simulink model "Exp01_06_Single_Phase_Transformer"  (R2023a)
settings: Solver=VariableStepAuto  StartTime=0.0  StopTime=.02  RelTol=1e-3
libraries: nesl_utility x13, fl_lib x8, ee_lib x8, spsPowerLib x2, spsRMSLib x2, spspowerguiLib x1
settings Model: Creator=dougs  LastModifiedBy=rafin
settings SolverCC: AlgebraicLoopSolver=TrustRegion
settings DebuggingCC: UnconnectedInputMsg=warning  UnconnectedOutputMsg=warning  UnconnectedLineMsg=warning
settings ModelReferenceCC: EnableRefExpFcnMdlSchedulingChecks=on
settings RTWCC: DLArmComputeVersion=19.05

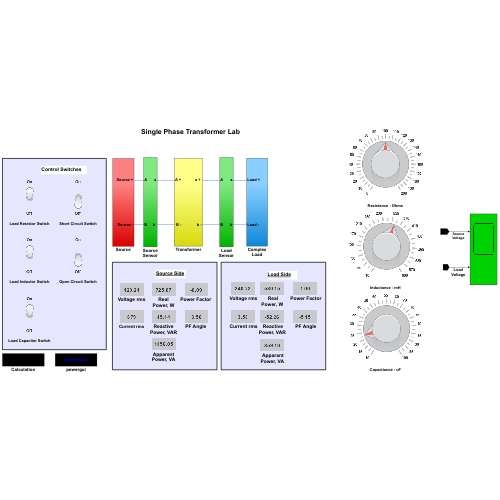
[thumbnail: Simulink's stored preview of the top-level diagram]
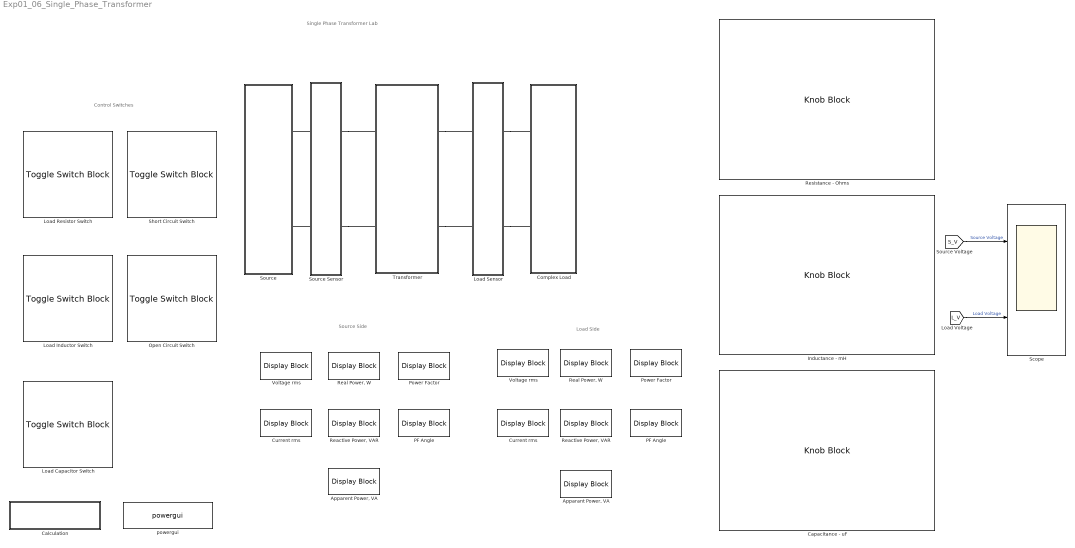
== system Exp01_06_Single_Phase_Transformer ==
  note: Control Switches
  note: Source Side
  note: Single Phase Transformer Lab
  note: Load Side
  " Apparant Power, VA" : DisplayBlock  LabelPosition=Hide  Format=bank  Transparency=1
  " Current rms" : DisplayBlock  LabelPosition=Hide  Format=bank  Transparency=1
  " PF Angle" : DisplayBlock  LabelPosition=Hide  Format=bank  Transparency=1
  " Power Factor" : DisplayBlock  LabelPosition=Hide  Format=bank  Transparency=1
  " Reactive Power, VAR" : DisplayBlock  LabelPosition=Hide  Format=bank  Transparency=1
  " Real Power, W" : DisplayBlock  LabelPosition=Hide  Format=bank  Transparency=1
  " Voltage rms" : DisplayBlock  LabelPosition=Hide  Format=bank  Transparency=1
  "Apparent Power, VA" : DisplayBlock  LabelPosition=Hide  Format=bank  Transparency=1
  Calculation : Subsystem
  Capacitance - uF : KnobBlock  LabelPosition=Hide  ScaleMin=10
  Complex Load : Subsystem
  Current rms : DisplayBlock  LabelPosition=Hide  Format=bank  Transparency=1
  Inductance - mH : KnobBlock  LabelPosition=Hide  ScaleMin=10  ScaleMax=600
  Load Sensor : Subsystem
  Load Capacitor Switch : ToggleSwitchBlock  LabelPosition=Hide
      settings: Values={{'Off', 'On'}, [0 2]}
  Load Inductor Switch : ToggleSwitchBlock  LabelPosition=Hide
      settings: Values={{'Off', 'On'}, [0 2]}
  Load Resistor Switch : ToggleSwitchBlock  LabelPosition=Hide
      settings: Values={{'Off', 'On'}, [0 2]}
  Open Circuit Switch : ToggleSwitchBlock  LabelPosition=Hide
      settings: Values={{'Off', 'On'}, [2 -2]}
  "PF Angle " : DisplayBlock  LabelPosition=Hide  Format=bank  Transparency=1
  "Power Factor " : DisplayBlock  LabelPosition=Hide  Format=bank  Transparency=1
  "Reactive Power, VAR" : DisplayBlock  LabelPosition=Hide  Format=bank  Transparency=1
  "Real Power, W" : DisplayBlock  LabelPosition=Hide  Format=bank  Transparency=1
  Resistance - Ohms : KnobBlock  LabelPosition=Hide  ScaleMax=200  TickInterval=10
  Scope : Scope  NumInputPorts=2
  Short Circuit Switch : ToggleSwitchBlock  LabelPosition=Hide
      settings: Values={{'Off', 'On'}, [0 2]}
  Source : Subsystem
      settings: PortSchema="{\"entries\":[{\"content\":{\"sides\":[{\"content\":{\"connectorIds\":[]},\"type\":\"ConnectorPlacement.EquallySpacedRectSide\",\"uuid\":\"e57deccf-7da9-425e-89f3-6f5e29807383\"},{\"content\":{\"connectorIds\":[],\"side\":\"RIGHT\"},\"type\":\"ConnectorPlacement.EquallySpacedRectSide\",\"uuid\":\"3e2a9798-8009-4f77-a4c3-5ae74279a04d\"},{\"content\":{\"connectorIds\":[],\"side\":\"TOP\"},\"type\":\"ConnectorPlacement.EquallySpacedRectSide\",\"uuid\":\"7dc73e5d-785d-4517-961f-ba0b2f479572\"},{\"content\":{\"connectorIds\":[\"RConn1\",\"RConn2\"],\"side\":\"BOTTOM\"},\"type\":\"ConnectorPlacement.EquallySpacedRectSide\",\"uuid\":\"c1959ef5-3070-4240-ae81-20c207906e41\"}]},\"type\":\"ConnectorPlacement.EquallySpacedConnector\",\"uuid\":\"719f97bd-ed7f-4cfa-8d10-4518bed19cde\"}],\"packageUris\":[\"http://schema.mathworks.com/mf0/Connector/R2020b\"],\"version\":\"1.0\"}"
  Source Sensor : Subsystem
  Transformer : Subsystem
  Voltage rms : DisplayBlock  LabelPosition=Hide  Format=bank  Transparency=1
  powergui : spspowerguiLib/powergui  Priority=1  SimulationMode=Continuous  SampleTime=50e-6  frequency=60  Iterations=50  frequencyindice=60  Pbase=100e6  ErrMax=1e-4  UnitsV=kV  UnitsW=MW  buscounter=0  FunctionMessages=off  echomessages=off  EnableUseOfTLC=off  CurrentSourceSwitches=off  DisableSnubberDevices=off  DisableRonSwitches=off  DisableVfSwitches=off  DisplayEquations=off  AutomaticDiscreteSolvers=off  SolverType=Tustin/Backward Euler (TBE)  Interpol=off  ExternalGateDelay=off  methode=off  Ts=100  x0status=blocks  SPID=on  SwTol=0  HookPort=off  NonlinearTolerance=1e-4  nMaxIteration=100  ContinueOnMaxIteration=off  RestoreLinks=warning  ResistiveCurrentMeasurement=off  Frange=[0:2:500]  Ylog=off  Xlog=on  ShowGrid=off  save=off  variable=ZData  structure=0  ZoomFFT=off  StartTime=0.0  cycles=1  DisplayStyle=1  fundamental=60  FreqAxis=off  MaxFrequency=1000  frequencyindicesteady=1  RmsSteady=1  display=off
  wires:
  [S_V] -> Scope/1  "Source Voltage"
  [L_V] -> Scope/2  "Load Voltage"
  connections:
  Load Sensor/RConn2 -- Complex Load/LConn2
  Load Sensor/RConn1 -- Complex Load/LConn1
  Transformer/RConn2 -- Load Sensor/LConn2
  Transformer/RConn1 -- Load Sensor/LConn1
  Source Sensor/RConn1 -- Transformer/LConn1
  Source Sensor/RConn2 -- Transformer/LConn2
  Source Sensor/LConn1 -- Source/RConn1
  Source Sensor/LConn2 -- Source/RConn2

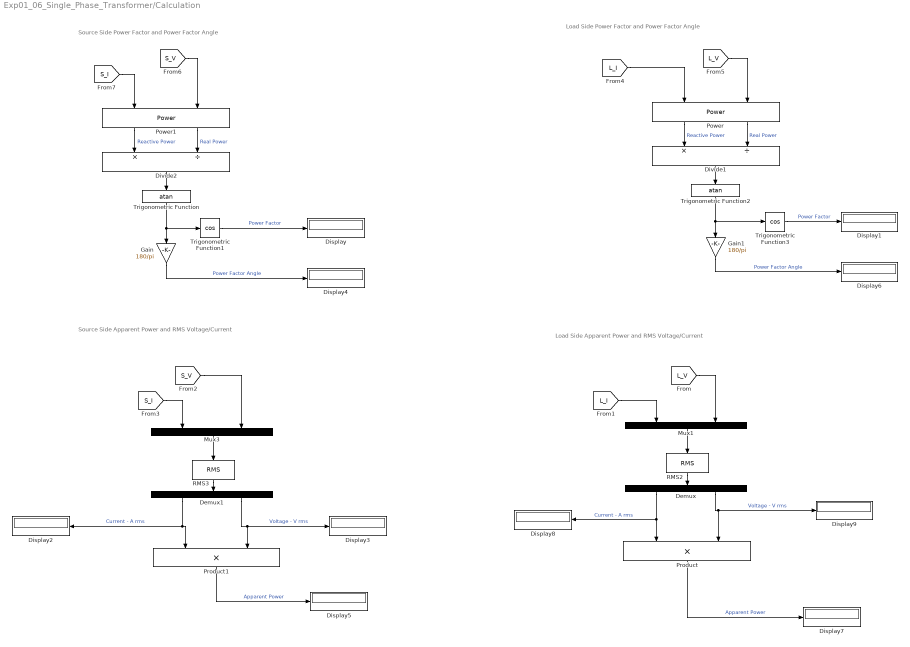
== system Exp01_06_Single_Phase_Transformer/Calculation ==
  note: Source Side Power Factor and Power Factor Angle
  note: Source Side Apparent Power and RMS Voltage/Current
  note: Load Side Power Factor and Power Factor Angle
  note: Load Side Apparent Power and RMS Voltage/Current
  Demux : Demux  Outputs=2
  Demux1 : Demux  Outputs=2
  Display{,1..9} (10 alike) : Display
  Divide1 : Product  Inputs=*/
  Divide2 : Product  Inputs=*/
  Gain : Gain  Gain=180/pi
  Gain1 : Gain  Gain=180/pi
  Mux1 : Mux  Inputs=2
  Mux3 : Mux  Inputs=2
  Power : spsPowerLib/Power  Freq=60  Vinit=[1, 0]  Iinit=[1, 0]  Ts=0
  Power1 : spsPowerLib/Power  Freq=60  Vinit=[1, 0]  Iinit=[1, 0]  Ts=0
  Product : Product
  Product1 : Product
  RMS2 : spsRMSLib/RMS  TrueRMS=on  Freq=60  RMSInit=120  Ts=0
  RMS3 : spsRMSLib/RMS  TrueRMS=on  Freq=60  RMSInit=120  Ts=0
  Trigonometric Function : Trigonometry  Operator=atan
  Trigonometric Function1 : Trigonometry  Operator=cos
  Trigonometric Function2 : Trigonometry  Operator=atan
  Trigonometric Function3 : Trigonometry  Operator=cos
  wires:
  [L_I] -> Mux1/1
  [L_V] -> Mux1/2
  Power/1 -> Divide1/2  "Real Power"
  Product/1 -> Display7/1  "Apparent Power"
  Power/2 -> Divide1/1  "Reactive Power"
  Mux1/1 -> RMS2/1
  [S_I] -> Mux3/1
  [S_V] -> Mux3/2
  Product1/1 -> Display5/1  "Apparent Power"
  Mux3/1 -> RMS3/1
  RMS3/1 -> Demux1/1
  Demux1/2 -> Product1/2, Display3/1  "Voltage - V rms"
  Demux1/1 -> Product1/1, Display2/1  "Current - A rms"
  [S_V] -> Power1/1
  [S_I] -> Power1/2
  Divide2/1 -> Trigonometric Function/1
  Trigonometric Function/1 -> Trigonometric Function1/1, Gain/1
  Gain/1 -> Display4/1  "Power Factor Angle"
  Power1/2 -> Divide2/1  "Reactive Power"
  Power1/1 -> Divide2/2  "Real Power"
  Trigonometric Function1/1 -> Display/1  "Power Factor"
  [L_V] -> Power/1
  [L_I] -> Power/2
  Divide1/1 -> Trigonometric Function2/1
  Trigonometric Function2/1 -> Gain1/1, Trigonometric Function3/1
  Trigonometric Function3/1 -> Display1/1  "Power Factor"
  Gain1/1 -> Display6/1  "Power Factor Angle"
  RMS2/1 -> Demux/1
  Demux/1 -> Product/1, Display8/1  "Current - A rms"
  Demux/2 -> Product/2, Display9/1  "Voltage - V rms"

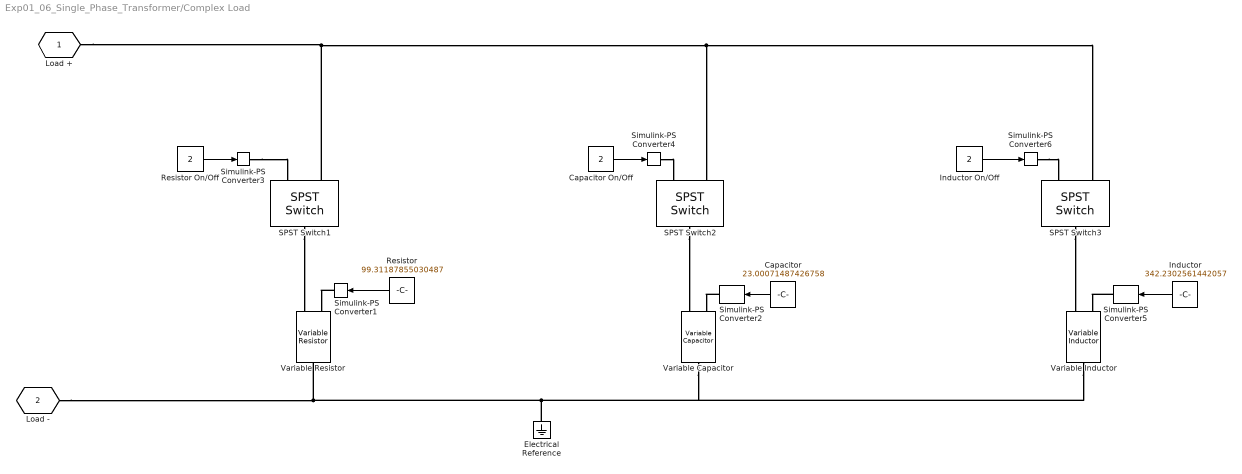
== system Exp01_06_Single_Phase_Transformer/Complex Load ==
  Capacitor : Constant  Value=23.00071487426758
  Capacitor On/Off : Constant  Value=2
  Electrical Reference : fl_lib/Electrical/Electrical Elements/Electrical Reference
  Inductor : Constant  Value=342.2302561442057
  Inductor On/Off : Constant  Value=2
  Resistor : Constant  Value=99.31187855030487
  Resistor On/Off : Constant  Value=2
  SPST Switch1 : ee_lib/Switches & Breakers/SPST Switch  R_closed=0.01 Ohm  G_open=1e-6 S  Threshold=1 V  Width=0 V  model_dynamics=0  t_on=1e-3 s  t_off=1e-3 s  initial_vT=0 V
      settings: InternalSimscapePortConfiguration="{\"Bottom\":[],\"Left\":[{\"id\":\"vT\",\"label\":\"vT\",\"type\":\"input\"},{\"id\":\"p\",\"label\":\"\",\"type\":\"foundation.electrical.electrical\"}],\"Right\":[{\"id\":\"n\",\"label\":\"\",\"type\":\"foundation.electrical.electrical\"}],\"Top\":[]}"
  SPST Switch2 : ee_lib/Switches & Breakers/SPST Switch  R_closed=0.01 Ohm  G_open=1e-6 S  Threshold=1 V  Width=0 V  model_dynamics=0  t_on=1e-3 s  t_off=1e-3 s  initial_vT=0 V
      settings: InternalSimscapePortConfiguration="{\"Bottom\":[],\"Left\":[{\"id\":\"vT\",\"label\":\"vT\",\"type\":\"input\"},{\"id\":\"p\",\"label\":\"\",\"type\":\"foundation.electrical.electrical\"}],\"Right\":[{\"id\":\"n\",\"label\":\"\",\"type\":\"foundation.electrical.electrical\"}],\"Top\":[]}"
  SPST Switch3 : ee_lib/Switches & Breakers/SPST Switch  R_closed=0.01 Ohm  G_open=1e-6 S  Threshold=1 V  Width=0 V  model_dynamics=0  t_on=1e-3 s  t_off=1e-3 s  initial_vT=0 V
      settings: InternalSimscapePortConfiguration="{\"Bottom\":[],\"Left\":[{\"id\":\"vT\",\"label\":\"vT\",\"type\":\"input\"},{\"id\":\"p\",\"label\":\"\",\"type\":\"foundation.electrical.electrical\"}],\"Right\":[{\"id\":\"n\",\"label\":\"\",\"type\":\"foundation.electrical.electrical\"}],\"Top\":[]}"
  Simulink-PS Converter1 : nesl_utility/Simulink-PS Converter  PhysicalDomain=network_engine_domain  SubClassName=ps_input  LeftPortType=input  RightPortType=output  PseudoPeriodic=off  Frequencies=[]  NoiseDistribution=none  NoiseParameters=[]  Unit=Ohm  AffineConversion=off  FilteringAndDerivatives=provide  SimscapeFilterOrder=1  InputFilterTimeConstant=0.001  UdotUserProvided=0
  Simulink-PS Converter2 : nesl_utility/Simulink-PS Converter  PhysicalDomain=network_engine_domain  SubClassName=ps_input  LeftPortType=input  RightPortType=output  PseudoPeriodic=off  Frequencies=[]  NoiseDistribution=none  NoiseParameters=[]  Unit=uF  AffineConversion=off  FilteringAndDerivatives=provide  SimscapeFilterOrder=1  InputFilterTimeConstant=0.001  UdotUserProvided=0
  Simulink-PS Converter3 : nesl_utility/Simulink-PS Converter  PhysicalDomain=network_engine_domain  SubClassName=ps_input  LeftPortType=input  RightPortType=output  PseudoPeriodic=off  Frequencies=[]  NoiseDistribution=none  NoiseParameters=[]  Unit=V  AffineConversion=off  FilteringAndDerivatives=provide  SimscapeFilterOrder=1  InputFilterTimeConstant=0.001  UdotUserProvided=0
  Simulink-PS Converter4 : nesl_utility/Simulink-PS Converter  PhysicalDomain=network_engine_domain  SubClassName=ps_input  LeftPortType=input  RightPortType=output  PseudoPeriodic=off  Frequencies=[]  NoiseDistribution=none  NoiseParameters=[]  Unit=V  AffineConversion=off  FilteringAndDerivatives=provide  SimscapeFilterOrder=1  InputFilterTimeConstant=0.001  UdotUserProvided=0
  Simulink-PS Converter5 : nesl_utility/Simulink-PS Converter  PhysicalDomain=network_engine_domain  SubClassName=ps_input  LeftPortType=input  RightPortType=output  PseudoPeriodic=off  Frequencies=[]  NoiseDistribution=none  NoiseParameters=[]  Unit=mH  AffineConversion=off  FilteringAndDerivatives=provide  SimscapeFilterOrder=1  InputFilterTimeConstant=0.001  UdotUserProvided=0
  Simulink-PS Converter6 : nesl_utility/Simulink-PS Converter  PhysicalDomain=network_engine_domain  SubClassName=ps_input  LeftPortType=input  RightPortType=output  PseudoPeriodic=off  Frequencies=[]  NoiseDistribution=none  NoiseParameters=[]  Unit=V  AffineConversion=off  FilteringAndDerivatives=provide  SimscapeFilterOrder=1  InputFilterTimeConstant=0.001  UdotUserProvided=0
  Variable Capacitor : ee_lib/Passive/Variable Capacitor  prm=2  Cmin=.000001 uF  r=1e-6 Ohm  v0=0 V  q0=0 C
      settings: InternalSimscapePortConfiguration="{\"Bottom\":[],\"Left\":[{\"id\":\"C\",\"label\":\"C\",\"type\":\"input\"},{\"id\":\"p\",\"label\":\"+\",\"type\":\"foundation.electrical.electrical\"}],\"Right\":[{\"id\":\"n\",\"label\":\"-\",\"type\":\"foundation.electrical.electrical\"}],\"Top\":[]}"
  Variable Inductor : ee_lib/Passive/Variable Inductor  prm=1  Lmin=1e-6 mH  g=1e-9 1/Ohm  i0=0 A  phi0=0 Wb
      settings: InternalSimscapePortConfiguration="{\"Bottom\":[],\"Left\":[{\"id\":\"L\",\"label\":\"L\",\"type\":\"input\"},{\"id\":\"p\",\"label\":\"+\",\"type\":\"foundation.electrical.electrical\"}],\"Right\":[{\"id\":\"n\",\"label\":\"-\",\"type\":\"foundation.electrical.electrical\"}],\"Top\":[]}"
  Variable Resistor : fl_lib/Electrical/Electrical Elements/Variable Resistor  Rmin=0 Ohm  i_specify=off  i_priority=None  i=23.72612403869629 A  i_nominal_specify=off  i_nominal_unit=A  i_nominal_value=1  v_specify=off  v_priority=None  v=0 V  v_nominal_specify=off  v_nominal_unit=V  v_nominal_value=1
  Load + : PMIOPort  Side=Left
  Load - : PMIOPort  Port=2  Side=Left
  wires:
  Capacitor/1 -> Simulink-PS Converter2/1
  Resistor/1 -> Simulink-PS Converter1/1
  Resistor On/Off/1 -> Simulink-PS Converter3/1
  Capacitor On/Off/1 -> Simulink-PS Converter4/1
  Inductor/1 -> Simulink-PS Converter5/1
  Inductor On/Off/1 -> Simulink-PS Converter6/1
  connections:
  Variable Inductor/RConn1 -- Variable Capacitor/RConn1 -- Electrical Reference/LConn1 -- Load -/RConn1 -- Variable Resistor/RConn1
  Simulink-PS Converter1/RConn1 -- Variable Resistor/LConn1
  Simulink-PS Converter2/RConn1 -- Variable Capacitor/LConn1
  Simulink-PS Converter3/RConn1 -- SPST Switch1/LConn1
  SPST Switch2/RConn1 -- Variable Capacitor/LConn2
  SPST Switch3/RConn1 -- Variable Inductor/LConn2
  SPST Switch1/LConn2 -- Load +/RConn1 -- SPST Switch2/LConn2 -- SPST Switch3/LConn2
  Simulink-PS Converter4/RConn1 -- SPST Switch2/LConn1
  SPST Switch1/RConn1 -- Variable Resistor/LConn2
  Simulink-PS Converter5/RConn1 -- Variable Inductor/LConn1
  Simulink-PS Converter6/RConn1 -- SPST Switch3/LConn1

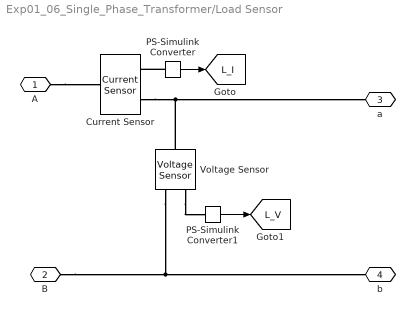
== system Exp01_06_Single_Phase_Transformer/Load Sensor ==
  Current Sensor : fl_lib/Electrical/Electrical Sensors/Current Sensor
  PS-Simulink Converter : nesl_utility/PS-Simulink Converter  PhysicalDomain=network_engine_domain  SubClassName=ps_output  LeftPortType=input  RightPortType=output  PseudoPeriodic=off  Frequencies=[]  VectorFormat=1-D array  Unit=inherit  AffineConversion=off
  PS-Simulink Converter1 : nesl_utility/PS-Simulink Converter  PhysicalDomain=network_engine_domain  SubClassName=ps_output  LeftPortType=input  RightPortType=output  PseudoPeriodic=off  Frequencies=[]  VectorFormat=1-D array  Unit=inherit  AffineConversion=off
  Voltage Sensor : fl_lib/Electrical/Electrical Sensors/Voltage Sensor
  "A " : PMIOPort  Side=Left
  B : PMIOPort  Port=2  Side=Left
  a : PMIOPort  Port=3  Side=Right
  b : PMIOPort  Port=4  Side=Right
  tag scope: L_I=global, L_V=global
  wires:
  PS-Simulink Converter/1 -> [L_I]
  PS-Simulink Converter1/1 -> [L_V]
  connections:
  Current Sensor/RConn2 -- a/RConn1 -- Voltage Sensor/LConn1
  Voltage Sensor/RConn2 -- b/RConn1 -- B/RConn1
  "A "/RConn1 -- Current Sensor/LConn1
  PS-Simulink Converter/LConn1 -- Current Sensor/RConn1
  Voltage Sensor/RConn1 -- PS-Simulink Converter1/LConn1

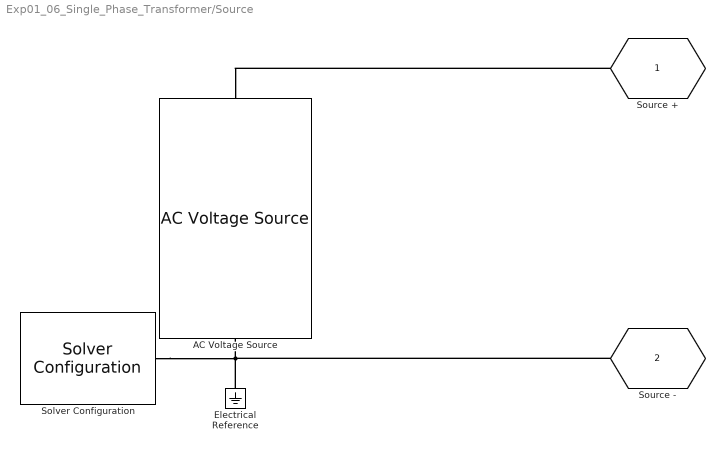
== system Exp01_06_Single_Phase_Transformer/Source ==
  AC Voltage Source : fl_lib/Electrical/Electrical Sources/AC Voltage Source  amp=170 V  shift=0 deg  frequency=60 Hz  omega=0 rad/s
  Electrical Reference : fl_lib/Electrical/Electrical Elements/Electrical Reference
  Solver Configuration : nesl_utility/Solver Configuration  PhysicalDomain=network_engine_domain  SubClassName=solver  LeftPortType=input  RightPortType=generic  Tones=[]  Harmonics=[]  SimulateNoise=off  Profile=off  UseLocalSampling=off  EnableSwitchedLinearOptims=on  FrequencyDomain=off  UseCCode=off  RelTol=0.001  AbsTol=1e-06  MinStep=1e-09  ToWorkspace=off  RevertToSquareIcSolve=off  NumHomotopyIterations=100  PhasorMode=off  PhasorModeNumHarmonics=1  ConsistencySolver=NEWTON_FTOL  IndexReductionMethod=DerivativeReplacement  DoDC=off  ResidualTolerance=1e-09  ConsistencyTolSource=GLOBAL  ConsistencyAbsTol=0.001  ConsistencyRelTol=0.001  ConsistencyTolFactor=0.001  UseLocalSolver=off  LocalSolverChoice=NE_BACKWARD_EULER_ADVANCER  ResolveIndetEquations=on  FunctionEvalNumThread=1  LocalSolverSampleTime=0.001  DoFixedCost=off  MaxNonlinIter=3  MaxModeIter=2  ComputeImpulses=off  ImpulseIterations=2  LinearAlgebra=auto  LinearAlgebraNumThread=0  EquationFormulation=NE_TIME_EF  DelaysMemoryBudget=1024  AutomaticFiltering=on  FilteringTimeConstant=0.001  PartitionStorageMethod=AS_NEEDED  PartitionMemoryBudget=1024  PartitionMethod=ROBUST
  Source + : PMIOPort  Side=Right
  Source - : PMIOPort  Port=2  Side=Right
  connections:
  Source -/RConn1 -- Electrical Reference/LConn1 -- Solver Configuration/RConn1 -- AC Voltage Source/RConn1
  Source +/RConn1 -- AC Voltage Source/LConn1

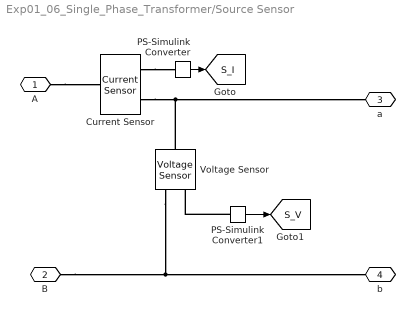
== system Exp01_06_Single_Phase_Transformer/Source Sensor ==
  Current Sensor : fl_lib/Electrical/Electrical Sensors/Current Sensor
  PS-Simulink Converter : nesl_utility/PS-Simulink Converter  PhysicalDomain=network_engine_domain  SubClassName=ps_output  LeftPortType=input  RightPortType=output  PseudoPeriodic=off  Frequencies=[]  VectorFormat=1-D array  Unit=inherit  AffineConversion=off
  PS-Simulink Converter1 : nesl_utility/PS-Simulink Converter  PhysicalDomain=network_engine_domain  SubClassName=ps_output  LeftPortType=input  RightPortType=output  PseudoPeriodic=off  Frequencies=[]  VectorFormat=1-D array  Unit=inherit  AffineConversion=off
  Voltage Sensor : fl_lib/Electrical/Electrical Sensors/Voltage Sensor
  "A " : PMIOPort  Side=Left
  B : PMIOPort  Port=2  Side=Left
  a : PMIOPort  Port=3  Side=Right
  "b " : PMIOPort  Port=4  Side=Right
  tag scope: S_I=global, S_V=global
  wires:
  PS-Simulink Converter/1 -> [S_I]
  PS-Simulink Converter1/1 -> [S_V]
  connections:
  Voltage Sensor/LConn1 -- Current Sensor/RConn2 -- a/RConn1
  B/RConn1 -- "b "/RConn1 -- Voltage Sensor/RConn2
  "A "/RConn1 -- Current Sensor/LConn1
  Current Sensor/RConn1 -- PS-Simulink Converter/LConn1
  PS-Simulink Converter1/LConn1 -- Voltage Sensor/RConn1

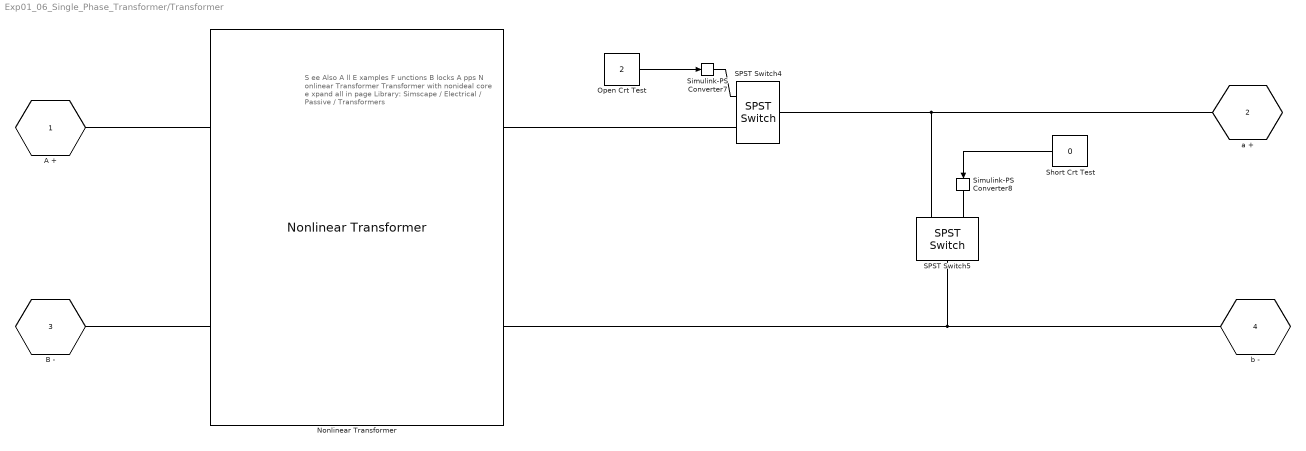
== system Exp01_06_Single_Phase_Transformer/Transformer ==
  note: S ee Also
      | A ll
      | E xamples
      | F unctions
      | B locks
      | A pps
      | N onlinear Transformer
      | Transformer with nonideal core
      | e xpand all in page
      | Library:
      | Simscape / Electrical / Passive / Transformers
  Nonlinear Transformer : ee_lib/Passive/Transformers/Nonlinear Transformer  Nw=100  Nw2=200  winding_param_option=2  Req=0.01 Ohm  Leq=0.0001 H  R_1=0.01 Ohm  L_1=0.0001 H  R_2=0.01 Ohm  L_2=0.0001 H  averaging_period=0 s  R_m=100 Ohm  parameterization_option=1  H_data=[0, 200, 400, 600, 800, 1000] A/m  B_data=[0, .81, 1.25, 1.42, 1.48, 1.49] T  length_effective=0.2 m  area_effective=2e-4 m^2  L=4e-1 H  L_sat=1e-2 H  current_data=[0, .4, .8, 1.2, 1.6, 2] A  magnetic_flux_data=[0, .161, .25, .284, .295, .299] .* 1e-3 Wb  magnetic_flux_sat=1.6e-04 Wb  dBdH0=0.005 m*T/A  B1=1.49 T  H1=1000 A/m  c=0.1  K=200 A/m  alpha=1e-4  interpolation_option=1  Leq_i0=0 A  L1_i0=0 A  L2_i0=0 A  x0_option=1  i_L0=0 A  phi0=0 Wb  B0=0 T  H0=0 A/m  Leq_g=1e-9 1/Ohm  L1_g=1e-9 1/Ohm  L2_g=1e-9 1/Ohm
      settings: InternalSimscapePortConfiguration="{\"Bottom\":[],\"Left\":[{\"id\":\"p1\",\"label\":\"1+\",\"type\":\"foundation.electrical.electrical\"},{\"id\":\"n1\",\"label\":\"1-\",\"type\":\"foundation.electrical.electrical\"}],\"Right\":[{\"id\":\"p2\",\"label\":\"2+\",\"type\":\"foundation.electrical.electrical\"},{\"id\":\"n2\",\"label\":\"2-\",\"type\":\"foundation.electrical.electrical\"}],\"Top\":[]}"
  Open Crt Test : Constant  Value=2
  SPST Switch4 : ee_lib/Switches & Breakers/SPST Switch  R_closed=0.0001 Ohm  G_open=1e-6 S  Threshold=1 V  Width=0 V  model_dynamics=0  t_on=1e-3 s  t_off=1e-3 s  initial_vT=0 V
      settings: InternalSimscapePortConfiguration="{\"Bottom\":[],\"Left\":[{\"id\":\"vT\",\"label\":\"vT\",\"type\":\"input\"},{\"id\":\"p\",\"label\":\"\",\"type\":\"foundation.electrical.electrical\"}],\"Right\":[{\"id\":\"n\",\"label\":\"\",\"type\":\"foundation.electrical.electrical\"}],\"Top\":[]}"
  SPST Switch5 : ee_lib/Switches & Breakers/SPST Switch  R_closed=0.000001 Ohm  G_open=1e-6 S  Threshold=1 V  Width=0 V  model_dynamics=0  t_on=1e-3 s  t_off=1e-3 s  initial_vT=0 V
      settings: InternalSimscapePortConfiguration="{\"Bottom\":[],\"Left\":[{\"id\":\"vT\",\"label\":\"vT\",\"type\":\"input\"},{\"id\":\"p\",\"label\":\"\",\"type\":\"foundation.electrical.electrical\"}],\"Right\":[{\"id\":\"n\",\"label\":\"\",\"type\":\"foundation.electrical.electrical\"}],\"Top\":[]}"
  Short Crt Test : Constant  Value=0
  Simulink-PS Converter7 : nesl_utility/Simulink-PS Converter  PhysicalDomain=network_engine_domain  SubClassName=ps_input  LeftPortType=input  RightPortType=output  PseudoPeriodic=off  Frequencies=[]  NoiseDistribution=none  NoiseParameters=[]  Unit=V  AffineConversion=off  FilteringAndDerivatives=provide  SimscapeFilterOrder=1  InputFilterTimeConstant=0.001  UdotUserProvided=0
  Simulink-PS Converter8 : nesl_utility/Simulink-PS Converter  PhysicalDomain=network_engine_domain  SubClassName=ps_input  LeftPortType=input  RightPortType=output  PseudoPeriodic=off  Frequencies=[]  NoiseDistribution=none  NoiseParameters=[]  Unit=V  AffineConversion=off  FilteringAndDerivatives=provide  SimscapeFilterOrder=1  InputFilterTimeConstant=0.001  UdotUserProvided=0
  A + : PMIOPort  Side=Left
  "a + " : PMIOPort  Port=2  Side=Right
  " B -" : PMIOPort  Port=3  Side=Left
  b - : PMIOPort  Port=4  Side=Right
  wires:
  Short Crt Test/1 -> Simulink-PS Converter8/1
  Open Crt Test/1 -> Simulink-PS Converter7/1
  connections:
  SPST Switch4/RConn1 -- SPST Switch5/LConn2 -- "a + "/RConn1
  A +/RConn1 -- Nonlinear Transformer/LConn1
  " B -"/RConn1 -- Nonlinear Transformer/LConn2
  b -/RConn1 -- SPST Switch5/RConn1 -- Nonlinear Transformer/RConn2
  Simulink-PS Converter8/RConn1 -- SPST Switch5/LConn1
  Simulink-PS Converter7/RConn1 -- SPST Switch4/LConn1
  Nonlinear Transformer/RConn1 -- SPST Switch4/LConn2
